simulink model "AUV_Plant"  (R2020a)
settings: Solver=VariableStepAuto  StartTime=0.0  StopTime=10.0  RelTol=1e-3
values from neighbouring files (symbols this model uses):
  a = [ 0 90 45 ... (first row only)    [plant_init.m]
undefined symbols (not defined in the file or in its folder): b, c
(part 1 of 2)
settings Model: Creator=Lamarre  LastModifiedBy=Lamarre

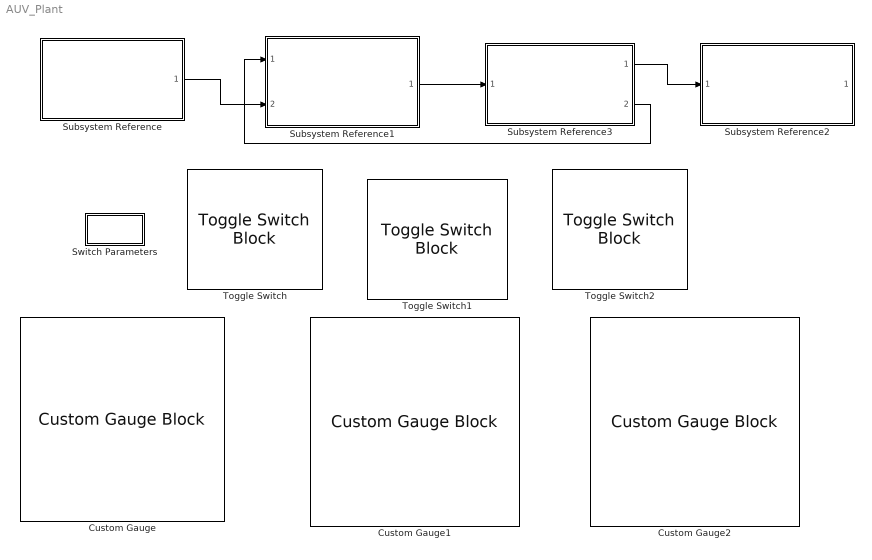
== system AUV_Plant ==
  Custom Gauge : CustomGaugeBlock  NeedleImage=data:image/svg+xml;base64,PD94bWwgdmVyc2lvbj0iMS4wIiBlbmNvZGluZz0idXRmLTgiPz4KPCEtLSBHZW5lcmF0b3I6IEFkb2JlIElsbHVzdHJhdG9yIDE5LjIuMSwgU1ZHIEV4cG9ydCBQbHVnLUluIC4gU1ZHIFZlcnNpb246IDYuMDAgQnVpbGQgMCkgIC0tPgo8c3ZnIHZlcnNpb249IjEuMSIgeG1sbnM9Imh0dHA6Ly93d3cudzMub3JnLzIwMDAvc3ZnIiB4bWxuczp4bGluaz0iaHR0cDovL3d3dy53My5vcmcvMTk5OS94bGluayIgeD0iMHB4IiB5PSIwcHgiCgkgdmlld0JveD0iMCAwIDIwMCA1MCIgc3R5bGU9ImVuYWJsZS1iYWNrZ3JvdW5kOm5ldyAw ...(+9940 chars)  NeedleXPos=0.37669652134625153  NeedleYPos=0.4806176508586912  NeedleHeight=0.11731129763666923  NeedleWidth=0.19326170036610194  NeedleInitialRotation=-59.94322499147643  BackgroundImage=data:image/svg+xml;base64,PD94bWwgdmVyc2lvbj0iMS4wIiBlbmNvZGluZz0iVVRGLTgiIHN0YW5kYWxvbmU9Im5vIj8+CjwhLS0gR2VuZXJhdG9yOiBBZG9iZSBJbGx1c3RyYXRvciAxOS4yLjEsIFNWRyBFeHBvcnQgUGx1Zy1JbiAuIFNWRyBWZXJzaW9uOiA2LjAwIEJ1aWxkIDApICAtLT4KCjxzdmcKICAgeG1sbnM6ZGM9Imh0dHA6Ly9wdXJsLm9yZy9kYy9lbGVtZW50cy8xLjEvIgogICB4bWxuczpjYz0iaHR0cDovL2NyZWF0aXZlY29tbW9ucy5vcmcvbnMjIgogICB4bWxuczpyZGY9Imh0dHA6Ly93d3cudzMub3JnLzE5OTkvMDIvMjItcmRmLXN5bnRh ...(+9660 chars)  GaugeMin=-1  GaugeMax=+1  GaugeArcDefined=true  GaugeArcRadius=0.1373666670427214  GaugeArcStrokeWidth=0.040171316096461976  GaugeArcRotation=240.5385250290321  GaugeArcRatio=0.8333333333333  GaugeArcTransparency=0  ValueArcColor=#1759b0  GaugeTickColor=#faf5c8  ScaleColorsJSON=[]  fixedAspectRatio=on  IsLinearGauge=false  GaugeTrackLeft=0.35  GaugeTrackTop=0.35  GaugeTrackHeight=0.1  GaugeTrackWidth=0.3  GaugeTrackRotation=0  ScaleMin=-1
  Custom Gauge1 : CustomGaugeBlock  NeedleImage=data:image/svg+xml;base64,PD94bWwgdmVyc2lvbj0iMS4wIiBlbmNvZGluZz0idXRmLTgiPz4KPCEtLSBHZW5lcmF0b3I6IEFkb2JlIElsbHVzdHJhdG9yIDE5LjIuMSwgU1ZHIEV4cG9ydCBQbHVnLUluIC4gU1ZHIFZlcnNpb246IDYuMDAgQnVpbGQgMCkgIC0tPgo8c3ZnIHZlcnNpb249IjEuMSIgeG1sbnM9Imh0dHA6Ly93d3cudzMub3JnLzIwMDAvc3ZnIiB4bWxuczp4bGluaz0iaHR0cDovL3d3dy53My5vcmcvMTk5OS94bGluayIgeD0iMHB4IiB5PSIwcHgiCgkgdmlld0JveD0iMCAwIDIwMCA1MCIgc3R5bGU9ImVuYWJsZS1iYWNrZ3JvdW5kOm5ldyAw ...(+9940 chars)  NeedleXPos=0.37838038678495906  NeedleYPos=0.48088234142700564  NeedleHeight=0.1157708144623717  NeedleWidth=0.19072386808866693  NeedleInitialRotation=-59.94322499147643  BackgroundImage=data:image/svg+xml;base64,PD94bWwgdmVyc2lvbj0iMS4wIiBlbmNvZGluZz0iVVRGLTgiIHN0YW5kYWxvbmU9Im5vIj8+CjwhLS0gR2VuZXJhdG9yOiBBZG9iZSBJbGx1c3RyYXRvciAxOS4yLjEsIFNWRyBFeHBvcnQgUGx1Zy1JbiAuIFNWRyBWZXJzaW9uOiA2LjAwIEJ1aWxkIDApICAtLT4KCjxzdmcKICAgeG1sbnM6ZGM9Imh0dHA6Ly9wdXJsLm9yZy9kYy9lbGVtZW50cy8xLjEvIgogICB4bWxuczpjYz0iaHR0cDovL2NyZWF0aXZlY29tbW9ucy5vcmcvbnMjIgogICB4bWxuczpyZGY9Imh0dHA6Ly93d3cudzMub3JnLzE5OTkvMDIvMjItcmRmLXN5bnRh ...(+9660 chars)  GaugeMin=-1  GaugeMax=+1  GaugeArcDefined=true  GaugeArcRadius=0.13556282509781314  GaugeArcStrokeWidth=0.039643803079534565  GaugeArcRotation=240.5385250290321  GaugeArcRatio=0.8333333333333  GaugeArcTransparency=0  ValueArcColor=#1759b0  GaugeTickColor=#faf5c8  ScaleColorsJSON=[]  fixedAspectRatio=on  IsLinearGauge=false  GaugeTrackLeft=0.35  GaugeTrackTop=0.35  GaugeTrackHeight=0.1  GaugeTrackWidth=0.3  GaugeTrackRotation=0  ScaleMin=-1
  Custom Gauge2 : CustomGaugeBlock  NeedleImage=data:image/svg+xml;base64,PD94bWwgdmVyc2lvbj0iMS4wIiBlbmNvZGluZz0idXRmLTgiPz4KPCEtLSBHZW5lcmF0b3I6IEFkb2JlIElsbHVzdHJhdG9yIDE5LjIuMSwgU1ZHIEV4cG9ydCBQbHVnLUluIC4gU1ZHIFZlcnNpb246IDYuMDAgQnVpbGQgMCkgIC0tPgo8c3ZnIHZlcnNpb249IjEuMSIgeG1sbnM9Imh0dHA6Ly93d3cudzMub3JnLzIwMDAvc3ZnIiB4bWxuczp4bGluaz0iaHR0cDovL3d3dy53My5vcmcvMTk5OS94bGluayIgeD0iMHB4IiB5PSIwcHgiCgkgdmlld0JveD0iMCAwIDIwMCA1MCIgc3R5bGU9ImVuYWJsZS1iYWNrZ3JvdW5kOm5ldyAw ...(+9940 chars)  NeedleXPos=0.3814875522631605  NeedleYPos=0.4813707637067003  NeedleHeight=0.1128130754220022  NeedleWidth=0.18585121142475902  NeedleInitialRotation=-59.94322499147643  BackgroundImage=data:image/svg+xml;base64,PD94bWwgdmVyc2lvbj0iMS4wIiBlbmNvZGluZz0iVVRGLTgiIHN0YW5kYWxvbmU9Im5vIj8+CjwhLS0gR2VuZXJhdG9yOiBBZG9iZSBJbGx1c3RyYXRvciAxOS4yLjEsIFNWRyBFeHBvcnQgUGx1Zy1JbiAuIFNWRyBWZXJzaW9uOiA2LjAwIEJ1aWxkIDApICAtLT4KCjxzdmcKICAgeG1sbnM6ZGM9Imh0dHA6Ly9wdXJsLm9yZy9kYy9lbGVtZW50cy8xLjEvIgogICB4bWxuczpjYz0iaHR0cDovL2NyZWF0aXZlY29tbW9ucy5vcmcvbnMjIgogICB4bWxuczpyZGY9Imh0dHA6Ly93d3cudzMub3JnLzE5OTkvMDIvMjItcmRmLXN5bnRh ...(+9660 chars)  GaugeMin=-1  GaugeMax=+1  GaugeArcDefined=true  GaugeArcRadius=0.1320994352782235  GaugeArcStrokeWidth=0.03863097420188018  GaugeArcRotation=240.5385250290321  GaugeArcRatio=0.8333333333333  GaugeArcTransparency=0  ValueArcColor=#1759b0  GaugeTickColor=#faf5c8  ScaleColorsJSON=[]  fixedAspectRatio=on  IsLinearGauge=false  GaugeTrackLeft=0.35  GaugeTrackTop=0.35  GaugeTrackHeight=0.1  GaugeTrackWidth=0.3  GaugeTrackRotation=0  ScaleMin=-1
  Subsystem Reference : Subsystem  ReferencedSubsystem=Sub_Reference_parameters
  Subsystem Reference1 : Subsystem  ReferencedSubsystem=Sub_Controller
  Subsystem Reference2 : Subsystem  ReferencedSubsystem=Sub_Sensor_Data
  Subsystem Reference3 : Subsystem  ReferencedSubsystem=Sub_Plant_and_Environment_Model
  Switch Parameters : Subsystem
      mask Display: text(0.5, 0.5, 'Switch Parameters', 'horizontalAlignment', 'center')
  Toggle Switch : ToggleSwitchBlock
      settings: Values={{'Velocity Control', 'Position Control'}, [1 0]}
  Toggle Switch1 : ToggleSwitchBlock
      settings: Values={{'Low Fidelity Simulation', 'High Fidelity Simulation'}, [0 1]}
  Toggle Switch2 : ToggleSwitchBlock
      settings: Values={{'System with Noise', 'System without Noise'}, [0 1]}
  wires:
  Subsystem Reference/1 -> Subsystem Reference1/2
  Subsystem Reference1/1 -> Subsystem Reference3/1
  Subsystem Reference3/1 -> Subsystem Reference2/1
  Subsystem Reference3/2 -> Subsystem Reference1/1
